simulink model "bulk_boost_eq"  (R2020b)
settings: Solver=VariableStepAuto  StartTime=0.0  StopTime=0.6  FixedStep=t_step
undefined symbols (not defined in the file): C_eq, Cb, k, ki_1, ki_bulk, kp_1, kp_bulk, L_eq, Lb, R_eq, Rb, t_step, Vl, Vs
libraries: powerlib x19, powerlib_meascontrol x5
settings Model: Creator=Chuanyue Li  LastModifiedBy=c2107789
settings DataIOCC: ReturnWorkspaceOutputs=off
settings DebuggingCC: ArithmeticOperatorsInVariantConditions=warning
settings SFSimCC: SimUseLocalCustomCode=off  CustomCodeUndefinedFunction=UseInterfaceOnly
settings RTWCC: RTWUseLocalCustomCode=off

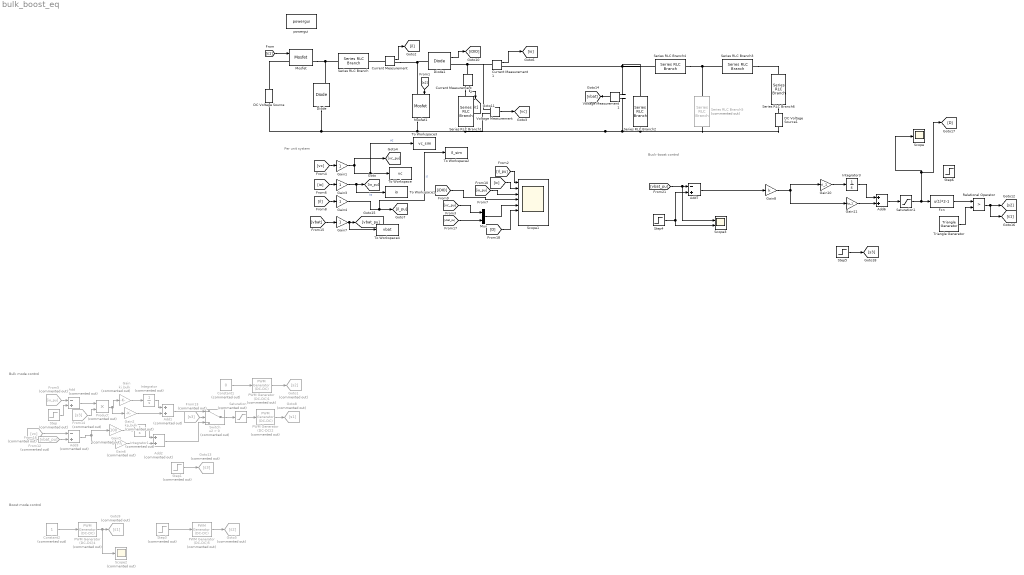
== system bulk_boost_eq ==
  note: Bulk mode control
  note: Per unit system
  note: Boost mode control
  note: Buck-boost control
  Add : Sum  Commented=on  Inputs=-+
  Add1 : Sum  Commented=on
  Add2 : Sum  Commented=on
  Add3 : Sum  Commented=on  Inputs=-+
  Add6 : Sum
  Add7 : Sum  Inputs=-+
  Constant1 : Constant  Commented=on  Value=0
  Constant2 : Constant  Commented=on
  Current Measurement : powerlib/Measurements/Current Measurement  PhasorSimulation=off  OutputType=Complex  PSBequivalent=0
  Current Measurement1 : powerlib/Measurements/Current Measurement  PhasorSimulation=off  OutputType=Complex  PSBequivalent=0
  Current Measurement2 : powerlib/Measurements/Current Measurement  PhasorSimulation=off  OutputType=Complex  PSBequivalent=0
  DC Voltage Source : powerlib/Electrical Sources/DC Voltage Source  Amplitude=Vs  Measurements=None
  DC Voltage Source1 : powerlib/Electrical Sources/DC Voltage Source  Amplitude=Vl  Measurements=None
  Diode : powerlib/Power Electronics/Diode  Ron=0.001  Lon=0  Vf=0  IC=0  UseSnubber=0  Rs=500000  Cs=250e-9  Measurements=on
  Diode1 : powerlib/Power Electronics/Diode  Ron=0.001  Lon=0  Vf=0  IC=0  UseSnubber=0  Rs=500000  Cs=250e-9  Measurements=on
  Fcn : Fcn  Expr=u(1)*2-1
  From12 : From  Commented=on  GotoTag=vc
  From13 : From  Commented=on  GotoTag=s3
  From14 : From  Commented=on  GotoTag=s3
  From16 : From  Commented=on  GotoTag=vbat_pu
  From5 : From  Commented=on  GotoTag=io_pu
  Gain : Gain  Commented=on  Gain=ki_bulk
  Gain{1,3..4,7} (4 alike) : Gain
  Gain10 : Gain  Gain=ki_1
  Gain11 : Gain  Gain=kp_1
  Gain2 : Gain  Commented=on  Gain=kp_bulk
  Gain5 : Gain  Commented=on  Gain=100
  Gain6 : Gain  Commented=on  Gain=0.1
  Gain8 : Gain  Gain=k
  Goto1 : Goto  Commented=on  GotoTag=s2
  Goto13 : Goto  Commented=on  GotoTag=s3
  Goto5 : Goto  Commented=on  GotoTag=s2
  Goto8 : Goto  Commented=on  GotoTag=s1
  Goto9 : Goto  Commented=on  GotoTag=s1
  Integrator : Integrator  Commented=on
  Integrator1 : Integrator  Commented=on
  Integrator3 : Integrator  InitialCondition=0.1
  Mosfet : powerlib/Power Electronics/Mosfet  Ron=0.01  Lon=0  Rd=0.01  Vfd=0  IC=0  Rs=1e5  Cs=inf  Measurements=on
  Mosfet1 : powerlib/Power Electronics/Mosfet  Ron=0.01  Lon=0  Rd=0.01  Vfd=0  IC=0  Rs=1e5  Cs=inf  Measurements=on
  Mux : Mux  Inputs=2
  PWM Generator (DC-DC){1..2,4..5} (4 alike) : powerlib_meascontrol/Pulse & Signal Generators/PWM Generator (DC-DC)  Commented=on  Fsw=s_fre  Ts=0
  Product : Product  Commented=on
  Relational Operator : RelationalOperator  Operator=>  OutDataTypeStr=boolean  RndMeth=Zero
  Saturation : Saturate  Commented=on  UpperLimit=1  LowerLimit=0
  Saturation1 : Saturate  UpperLimit=0.95  LowerLimit=-0.95
  Scope : Scope
  Scope1 : Scope  NumInputPorts=8
  Scope2 : Scope  Commented=on
  Scope3 : Scope  NumInputPorts=2
  Series RLC Branch : powerlib/Elements/Series RLC Branch  LConnTagsString=__new0  RConnTagsString=__new0  BranchType=L  Resistance=1  Inductance=Lb  SetiL0=off  InitialCurrent=0  Capacitance=1e-6  Setx0=off  InitialVoltage=0  Measurements=None
  Series RLC Branch1 : powerlib/Elements/Series RLC Branch  LConnTagsString=__new0  RConnTagsString=__new0  BranchType=C  Resistance=1  Inductance=1e-3  SetiL0=off  InitialCurrent=0  Capacitance=Cb  Setx0=off  InitialVoltage=0  Measurements=None
  Series RLC Branch2 : powerlib/Elements/Series RLC Branch  LConnTagsString=__new0  RConnTagsString=__new0  BranchType=C  Resistance=1  Inductance=1e-3  SetiL0=off  InitialCurrent=0  Capacitance=C_eq  Setx0=off  InitialVoltage=0  Measurements=None
  Series RLC Branch3 : powerlib/Elements/Series RLC Branch  LConnTagsString=__new0  RConnTagsString=__new0  BranchType=R  Resistance=R_eq  Inductance=Lb  SetiL0=off  InitialCurrent=0  Capacitance=1e-6  Setx0=off  InitialVoltage=0  Measurements=None
  Series RLC Branch4 : powerlib/Elements/Series RLC Branch  LConnTagsString=__new0  RConnTagsString=__new0  BranchType=L  Resistance=1  Inductance=L_eq  SetiL0=off  InitialCurrent=0  Capacitance=1e-6  Setx0=off  InitialVoltage=0  Measurements=None
  Series RLC Branch5 : powerlib/Elements/Series RLC Branch  Commented=on  LConnTagsString=__new0  RConnTagsString=__new0  BranchType=R  Resistance=Rb*400  Inductance=Lb  SetiL0=off  InitialCurrent=0  Capacitance=1e-6  Setx0=off  InitialVoltage=0  Measurements=None
  Series RLC Branch6 : powerlib/Elements/Series RLC Branch  LConnTagsString=__new0  RConnTagsString=__new0  BranchType=R  Resistance=Rb  Inductance=Lb  SetiL0=off  InitialCurrent=0  Capacitance=1e-6  Setx0=off  InitialVoltage=0  Measurements=None
  Step : Step  Commented=on  Time=0.1  Before=1  After=1.1  SampleTime=0
  Step1 : Step  Commented=on  Time=0.05  SampleTime=0
  Step3 : Step  Commented=on  Time=0.1  Before=0.9  After=0.9  SampleTime=0
  Step4 : Step  Time=0.4  Before=410  After=415  SampleTime=0
  Step5 : Step  Time=0.05  Before=1  SampleTime=0
  Step6 : Step  Time=0.3  Before=0.1  After=0.15  SampleTime=0
  Switch : Switch  Commented=on  Criteria=u2 > Threshold
  To Workspace : ToWorkspace  VariableName=vc  SaveFormat=Timeseries  SampleTime=-1
  To Workspace1 : ToWorkspace  VariableName=io  SaveFormat=Timeseries  SampleTime=-1
  To Workspace2 : ToWorkspace  VariableName=Il_sim  SaveFormat=Timeseries  SampleTime=-1
  To Workspace3 : ToWorkspace  VariableName=vc_sim  SaveFormat=Timeseries  SampleTime=-1
  To Workspace4 : ToWorkspace  VariableName=vbat  SaveFormat=Timeseries  SampleTime=-1
  Triangle Generator : powerlib_meascontrol/Pulse & Signal Generators/Triangle Generator  Freq=s_fre  Phase=0  Ts=0
  Voltage Measurement : powerlib/Measurements/Voltage Measurement  PhasorSimulation=off  OutputType=Complex  PSBequivalent=0
  Voltage Measurement1 : powerlib/Measurements/Voltage Measurement  PhasorSimulation=off  OutputType=Complex  PSBequivalent=0
  powergui : powerlib/powergui  Priority=1  SimulationMode=Continuous  SampleTime=t_step  frequency=60  Iterations=50  frequencyindice=0  Pbase=100e6  ErrMax=1e-4  UnitsV=kV  UnitsW=MW  buscounter=0  FunctionMessages=off  echomessages=off  EnableUseOfTLC=off  CurrentSourceSwitches=off  DisableSnubberDevices=off  DisableRonSwitches=off  DisableVfSwitches=off  DisplayEquations=off  AutomaticDiscreteSolvers=off  SolverType=Tustin/Backward Euler (TBE)  Interpol=off  ExternalGateDelay=off  methode=off  Ts=100  x0status=blocks  SPID=off  SwTol=0  HookPort=off  NonlinearTolerance=1e-4  nMaxIteration=100  ContinueOnMaxIteration=off  RestoreLinks=warning  ResistiveCurrentMeasurement=off  Frange=[0:2:500]  Ylog=off  Xlog=on  ShowGrid=off  save=off  variable=ZData  structure=logsout  ZoomFFT=off  StartTime=0.2  cycles=10  DisplayStyle=2  fundamental=50  FreqAxis=off  MaxFrequency=1000  frequencyindicesteady=1  RmsSteady=1  display=off
  wires:
  [s1] -> Mosfet/1
  Constant1/1 -> PWM Generator (DC-DC)1/1
  [s2] -> Mosfet1/1
  PWM Generator (DC-DC)1/1 -> Goto1/1
  Current Measurement/1 -> [il]
  Voltage Measurement/1 -> [vc]
  [il_pu] -> Scope1/1
  [vc] -> Gain1/1
  Gain1/1 -> To Workspace3/1, To Workspace/1, [vc_pu]  "vc"
  From5/1 -> Add/1
  Step/1 -> Add/2
  Gain/1 -> Integrator/1
  Integrator/1 -> Add1/1
  Saturation/1 -> PWM Generator (DC-DC)2/1
  PWM Generator (DC-DC)2/1 -> Goto8/1
  [io] -> Gain3/1
  Current Measurement1/1 -> [io]
  Gain3/1 -> To Workspace1/1, [io_pu]  "io"
  [io_pu] -> Scope1/3
  Gain2/1 -> Add1/2
  Gain4/1 -> To Workspace2/1, [il_pu]  "il"
  [il] -> Gain4/1
  Step3/1 -> PWM Generator (DC-DC)5/1
  Constant2/1 -> PWM Generator (DC-DC)4/1
  PWM Generator (DC-DC)4/1 -> Scope2/1, Goto9/1
  PWM Generator (DC-DC)5/1 -> Goto5/1
  Diode1/1 -> [iDIO]
  [iDIO] -> Scope1/4
  Current Measurement2/1 -> [ic]
  [ic] -> Scope1/2
  Add1/1 -> Switch/1
  Switch/1 -> Saturation/1
  Gain6/1 -> Add2/2
  Gain5/1 -> Integrator1/1
  Add3/1 -> Gain6/1, Gain5/1
  Add2/1 -> Switch/3
  Integrator1/1 -> Add2/1
  From12/1 -> Add3/1
  Step1/1 -> Goto13/1
  From13/1 -> Switch/2
  Add/1 -> Product/1
  Product/1 -> Gain2/1, Gain/1
  From14/1 -> Product/2
  Voltage Measurement1/1 -> [vbat]
  [vbat] -> Gain7/1
  Gain7/1 -> To Workspace4/1, [vbat_pu]
  From16/1 -> Add3/2
  [vc_pu] -> Mux/1
  Mux/1 -> Scope1/5
  [vbat_pu] -> Mux/2
  Triangle Generator/1 -> Relational Operator/2
  Fcn/1 -> Relational Operator/1
  Relational Operator/1 -> [s1], [s2]
  Step5/1 -> [s3]
  Add6/1 -> Saturation1/1
  Integrator3/1 -> Add6/1
  Gain11/1 -> Add6/2
  Saturation1/1 -> [D], Scope/1, Fcn/1
  [vbat_pu] -> Scope3/1, Add7/1
  Gain10/1 -> Integrator3/1
  Gain8/1 -> Gain11/1, Gain10/1
  Step4/1 -> Add7/2, Scope3/2
  [D] -> Scope1/6
  Add7/1 -> Gain8/1
  connections:
  DC Voltage Source/RConn1 -- Mosfet/LConn1
  Mosfet/RConn1 -- Diode/RConn1 -- Series RLC Branch/LConn1
  Mosfet1/LConn1 -- Current Measurement/RConn1 -- Diode1/LConn1
  Diode/LConn1 -- DC Voltage Source/LConn1 -- Voltage Measurement/LConn2 -- DC Voltage Source1/LConn1 -- Series RLC Branch5/LConn1 -- Series RLC Branch2/RConn1 -- Voltage Measurement1/LConn2 -- Series RLC Branch1/RConn1 -- Mosfet1/RConn1
  Current Measurement1/LConn1 -- Voltage Measurement/LConn1 -- Current Measurement2/LConn1 -- Diode1/RConn1
  Current Measurement/LConn1 -- Series RLC Branch/RConn1
  Current Measurement2/RConn1 -- Series RLC Branch1/LConn1
  Series RLC Branch3/LConn1 -- Series RLC Branch6/LConn1
  Voltage Measurement1/LConn1 -- Current Measurement1/RConn1 -- Series RLC Branch4/RConn1 -- Series RLC Branch2/LConn1
  Series RLC Branch4/LConn1 -- Series RLC Branch3/RConn1 -- Series RLC Branch5/RConn1
  Series RLC Branch6/RConn1 -- DC Voltage Source1/RConn1
